simulink model "MCity_cs"  (Simulink 8.9)
settings: Solver=ode5  StartTime=0.0  StopTime=3.95  FixedStep=1/200  RelTol=1e-3
PreLoadFcn:
  | check_NUTS_defined;
  | 
  | assignin('base',['model_closed_' bdroot],false);
InitFcn:
  | PreScanExperimentInitFcn(bdroot)
StopFcn:
  | PreScanExperimentStopFcn(bdroot)
values from neighbouring files (symbols this model uses):
  d_offset = -18.15    [monocityTestLeftTurn.mat]    (also in simulation_leftTurn_PreScan.m = dl/vl*vh - 43 + R)
undefined symbols (not defined in the file or in its folder): DiscIntNeverNeededParam, warningInitialVelocity, x0
libraries: simulink x78, PreScanSimulinkLibrary x14, simulink_extras x10, PreScanUsefulBlocks x4
(part 3 of 12)

== system MCity_cs/VISUCasingLights_1_TrafficLightDoubleUS_9 ==
  CasingLights : Inport
  Demux4 : Demux  Outputs=3
  Saturation1 : Saturate  UpperLimit=1  LowerLimit=0
  Saturation2 : Saturate  UpperLimit=1  LowerLimit=0
  Saturation3 : Saturate  UpperLimit=1  LowerLimit=0
  conv_Green : Subsystem
  conv_Orange : Subsystem
  conv_Red : Subsystem
  visu_CasingGreen : Subsystem  mask(ToSensorWorld){PortName=visu_LightCasingGreen_1, PortIndex=702, PortWidth=16, TimeStep=1/200}
      mask prompts: PortName "Port Name [-]"; PortIndex "Index [-]"; PortWidth "Port Dimensions [-]"; TimeStep "Upload Period [s]"
      mask help: Sends signal(s) from Simulink to the Sensor World
      mask Help:
      | Sends signal(s) from Simulink to the Sensor World.
      | 
      | - Port Name [-]: specifies the name of the output terminal of the Simulink block.
      | - Index [-]: specifies the start position in the output vector sent to the Sensor World
      | - Port dimensions [-]: specifies the width (number of scalars) of the output port
      | - Upload period [s]: specifies the upload period (in seconds) of the port.
      mask Display: port_label('input', 1, PortName)
  visu_CasingOrange : Subsystem  mask(ToSensorWorld){PortName=visu_LightCasingOrange_1, PortIndex=718, PortWidth=16, TimeStep=1/200}
      mask prompts: PortName "Port Name [-]"; PortIndex "Index [-]"; PortWidth "Port Dimensions [-]"; TimeStep "Upload Period [s]"
      mask help: Sends signal(s) from Simulink to the Sensor World
      mask Help:
      | Sends signal(s) from Simulink to the Sensor World.
      | 
      | - Port Name [-]: specifies the name of the output terminal of the Simulink block.
      | - Index [-]: specifies the start position in the output vector sent to the Sensor World
      | - Port dimensions [-]: specifies the width (number of scalars) of the output port
      | - Upload period [s]: specifies the upload period (in seconds) of the port.
      mask Display: port_label('input', 1, PortName)
  visu_CasingRed : Subsystem  mask(ToSensorWorld){PortName=visu_LightCasingRed_1, PortIndex=734, PortWidth=16, TimeStep=1/200}
      mask prompts: PortName "Port Name [-]"; PortIndex "Index [-]"; PortWidth "Port Dimensions [-]"; TimeStep "Upload Period [s]"
      mask help: Sends signal(s) from Simulink to the Sensor World
      mask Help:
      | Sends signal(s) from Simulink to the Sensor World.
      | 
      | - Port Name [-]: specifies the name of the output terminal of the Simulink block.
      | - Index [-]: specifies the start position in the output vector sent to the Sensor World
      | - Port dimensions [-]: specifies the width (number of scalars) of the output port
      | - Upload period [s]: specifies the upload period (in seconds) of the port.
      mask Display: port_label('input', 1, PortName)
  wires:
  CasingLights/1 -> Demux4/1
  Demux4/3 -> Saturation3/1
  Demux4/2 -> Saturation2/1
  Demux4/1 -> Saturation1/1
  Saturation1/1 -> conv_Red/1(on_off)
  Saturation2/1 -> conv_Orange/1(on_off)
  Saturation3/1 -> conv_Green/1(on_off)
  conv_Red/1(RGBcolor) -> visu_CasingRed/1(Y)
  conv_Orange/1(RGBcolor) -> visu_CasingOrange/1(Y)
  conv_Green/1(RGBcolor) -> visu_CasingGreen/1(Y)

== system MCity_cs/VISUCasingLights_2_TrafficLightDoubleUS_1 ==
  CasingLights : Inport
  Demux4 : Demux  Outputs=3
  Saturation1 : Saturate  UpperLimit=1  LowerLimit=0
  Saturation2 : Saturate  UpperLimit=1  LowerLimit=0
  Saturation3 : Saturate  UpperLimit=1  LowerLimit=0
  conv_Green : Subsystem
  conv_Orange : Subsystem
  conv_Red : Subsystem
  visu_CasingGreen : Subsystem  mask(ToSensorWorld){PortName=visu_LightCasingGreen_2, PortIndex=78, PortWidth=16, TimeStep=1/200}
      mask prompts: PortName "Port Name [-]"; PortIndex "Index [-]"; PortWidth "Port Dimensions [-]"; TimeStep "Upload Period [s]"
      mask help: Sends signal(s) from Simulink to the Sensor World
      mask Help:
      | Sends signal(s) from Simulink to the Sensor World.
      | 
      | - Port Name [-]: specifies the name of the output terminal of the Simulink block.
      | - Index [-]: specifies the start position in the output vector sent to the Sensor World
      | - Port dimensions [-]: specifies the width (number of scalars) of the output port
      | - Upload period [s]: specifies the upload period (in seconds) of the port.
      mask Display: port_label('input', 1, PortName)
  visu_CasingOrange : Subsystem  mask(ToSensorWorld){PortName=visu_LightCasingOrange_2, PortIndex=94, PortWidth=16, TimeStep=1/200}
      mask prompts: PortName "Port Name [-]"; PortIndex "Index [-]"; PortWidth "Port Dimensions [-]"; TimeStep "Upload Period [s]"
      mask help: Sends signal(s) from Simulink to the Sensor World
      mask Help:
      | Sends signal(s) from Simulink to the Sensor World.
      | 
      | - Port Name [-]: specifies the name of the output terminal of the Simulink block.
      | - Index [-]: specifies the start position in the output vector sent to the Sensor World
      | - Port dimensions [-]: specifies the width (number of scalars) of the output port
      | - Upload period [s]: specifies the upload period (in seconds) of the port.
      mask Display: port_label('input', 1, PortName)
  visu_CasingRed : Subsystem  mask(ToSensorWorld){PortName=visu_LightCasingRed_2, PortIndex=110, PortWidth=16, TimeStep=1/200}
      mask prompts: PortName "Port Name [-]"; PortIndex "Index [-]"; PortWidth "Port Dimensions [-]"; TimeStep "Upload Period [s]"
      mask help: Sends signal(s) from Simulink to the Sensor World
      mask Help:
      | Sends signal(s) from Simulink to the Sensor World.
      | 
      | - Port Name [-]: specifies the name of the output terminal of the Simulink block.
      | - Index [-]: specifies the start position in the output vector sent to the Sensor World
      | - Port dimensions [-]: specifies the width (number of scalars) of the output port
      | - Upload period [s]: specifies the upload period (in seconds) of the port.
      mask Display: port_label('input', 1, PortName)
  wires:
  CasingLights/1 -> Demux4/1
  Demux4/3 -> Saturation3/1
  Demux4/2 -> Saturation2/1
  Demux4/1 -> Saturation1/1
  Saturation1/1 -> conv_Red/1(on_off)
  Saturation2/1 -> conv_Orange/1(on_off)
  Saturation3/1 -> conv_Green/1(on_off)
  conv_Red/1(RGBcolor) -> visu_CasingRed/1(Y)
  conv_Orange/1(RGBcolor) -> visu_CasingOrange/1(Y)
  conv_Green/1(RGBcolor) -> visu_CasingGreen/1(Y)

== system MCity_cs/VISUCasingLights_2_TrafficLightDoubleUS_10 ==
  CasingLights : Inport
  Demux4 : Demux  Outputs=3
  Saturation1 : Saturate  UpperLimit=1  LowerLimit=0
  Saturation2 : Saturate  UpperLimit=1  LowerLimit=0
  Saturation3 : Saturate  UpperLimit=1  LowerLimit=0
  conv_Green : Subsystem
  conv_Orange : Subsystem
  conv_Red : Subsystem
  visu_CasingGreen : Subsystem  mask(ToSensorWorld){PortName=visu_LightCasingGreen_2, PortIndex=846, PortWidth=16, TimeStep=1/200}
      mask prompts: PortName "Port Name [-]"; PortIndex "Index [-]"; PortWidth "Port Dimensions [-]"; TimeStep "Upload Period [s]"
      mask help: Sends signal(s) from Simulink to the Sensor World
      mask Help:
      | Sends signal(s) from Simulink to the Sensor World.
      | 
      | - Port Name [-]: specifies the name of the output terminal of the Simulink block.
      | - Index [-]: specifies the start position in the output vector sent to the Sensor World
      | - Port dimensions [-]: specifies the width (number of scalars) of the output port
      | - Upload period [s]: specifies the upload period (in seconds) of the port.
      mask Display: port_label('input', 1, PortName)
  visu_CasingOrange : Subsystem  mask(ToSensorWorld){PortName=visu_LightCasingOrange_2, PortIndex=862, PortWidth=16, TimeStep=1/200}
      mask prompts: PortName "Port Name [-]"; PortIndex "Index [-]"; PortWidth "Port Dimensions [-]"; TimeStep "Upload Period [s]"
      mask help: Sends signal(s) from Simulink to the Sensor World
      mask Help:
      | Sends signal(s) from Simulink to the Sensor World.
      | 
      | - Port Name [-]: specifies the name of the output terminal of the Simulink block.
      | - Index [-]: specifies the start position in the output vector sent to the Sensor World
      | - Port dimensions [-]: specifies the width (number of scalars) of the output port
      | - Upload period [s]: specifies the upload period (in seconds) of the port.
      mask Display: port_label('input', 1, PortName)
  visu_CasingRed : Subsystem  mask(ToSensorWorld){PortName=visu_LightCasingRed_2, PortIndex=878, PortWidth=16, TimeStep=1/200}
      mask prompts: PortName "Port Name [-]"; PortIndex "Index [-]"; PortWidth "Port Dimensions [-]"; TimeStep "Upload Period [s]"
      mask help: Sends signal(s) from Simulink to the Sensor World
      mask Help:
      | Sends signal(s) from Simulink to the Sensor World.
      | 
      | - Port Name [-]: specifies the name of the output terminal of the Simulink block.
      | - Index [-]: specifies the start position in the output vector sent to the Sensor World
      | - Port dimensions [-]: specifies the width (number of scalars) of the output port
      | - Upload period [s]: specifies the upload period (in seconds) of the port.
      mask Display: port_label('input', 1, PortName)
  wires:
  CasingLights/1 -> Demux4/1
  Demux4/3 -> Saturation3/1
  Demux4/2 -> Saturation2/1
  Demux4/1 -> Saturation1/1
  Saturation1/1 -> conv_Red/1(on_off)
  Saturation2/1 -> conv_Orange/1(on_off)
  Saturation3/1 -> conv_Green/1(on_off)
  conv_Red/1(RGBcolor) -> visu_CasingRed/1(Y)
  conv_Orange/1(RGBcolor) -> visu_CasingOrange/1(Y)
  conv_Green/1(RGBcolor) -> visu_CasingGreen/1(Y)

== system MCity_cs/VISUCasingLights_2_TrafficLightDoubleUS_2 ==
  CasingLights : Inport
  Demux4 : Demux  Outputs=3
  Saturation1 : Saturate  UpperLimit=1  LowerLimit=0
  Saturation2 : Saturate  UpperLimit=1  LowerLimit=0
  Saturation3 : Saturate  UpperLimit=1  LowerLimit=0
  conv_Green : Subsystem
  conv_Orange : Subsystem
  conv_Red : Subsystem
  visu_CasingGreen : Subsystem  mask(ToSensorWorld){PortName=visu_LightCasingGreen_2, PortIndex=174, PortWidth=16, TimeStep=1/200}
      mask prompts: PortName "Port Name [-]"; PortIndex "Index [-]"; PortWidth "Port Dimensions [-]"; TimeStep "Upload Period [s]"
      mask help: Sends signal(s) from Simulink to the Sensor World
      mask Help:
      | Sends signal(s) from Simulink to the Sensor World.
      | 
      | - Port Name [-]: specifies the name of the output terminal of the Simulink block.
      | - Index [-]: specifies the start position in the output vector sent to the Sensor World
      | - Port dimensions [-]: specifies the width (number of scalars) of the output port
      | - Upload period [s]: specifies the upload period (in seconds) of the port.
      mask Display: port_label('input', 1, PortName)
  visu_CasingOrange : Subsystem  mask(ToSensorWorld){PortName=visu_LightCasingOrange_2, PortIndex=190, PortWidth=16, TimeStep=1/200}
      mask prompts: PortName "Port Name [-]"; PortIndex "Index [-]"; PortWidth "Port Dimensions [-]"; TimeStep "Upload Period [s]"
      mask help: Sends signal(s) from Simulink to the Sensor World
      mask Help:
      | Sends signal(s) from Simulink to the Sensor World.
      | 
      | - Port Name [-]: specifies the name of the output terminal of the Simulink block.
      | - Index [-]: specifies the start position in the output vector sent to the Sensor World
      | - Port dimensions [-]: specifies the width (number of scalars) of the output port
      | - Upload period [s]: specifies the upload period (in seconds) of the port.
      mask Display: port_label('input', 1, PortName)
  visu_CasingRed : Subsystem  mask(ToSensorWorld){PortName=visu_LightCasingRed_2, PortIndex=206, PortWidth=16, TimeStep=1/200}
      mask prompts: PortName "Port Name [-]"; PortIndex "Index [-]"; PortWidth "Port Dimensions [-]"; TimeStep "Upload Period [s]"
      mask help: Sends signal(s) from Simulink to the Sensor World
      mask Help:
      | Sends signal(s) from Simulink to the Sensor World.
      | 
      | - Port Name [-]: specifies the name of the output terminal of the Simulink block.
      | - Index [-]: specifies the start position in the output vector sent to the Sensor World
      | - Port dimensions [-]: specifies the width (number of scalars) of the output port
      | - Upload period [s]: specifies the upload period (in seconds) of the port.
      mask Display: port_label('input', 1, PortName)
  wires:
  CasingLights/1 -> Demux4/1
  Demux4/3 -> Saturation3/1
  Demux4/2 -> Saturation2/1
  Demux4/1 -> Saturation1/1
  Saturation1/1 -> conv_Red/1(on_off)
  Saturation2/1 -> conv_Orange/1(on_off)
  Saturation3/1 -> conv_Green/1(on_off)
  conv_Red/1(RGBcolor) -> visu_CasingRed/1(Y)
  conv_Orange/1(RGBcolor) -> visu_CasingOrange/1(Y)
  conv_Green/1(RGBcolor) -> visu_CasingGreen/1(Y)

== system MCity_cs/VISUCasingLights_2_TrafficLightDoubleUS_3 ==
  CasingLights : Inport
  Demux4 : Demux  Outputs=3
  Saturation1 : Saturate  UpperLimit=1  LowerLimit=0
  Saturation2 : Saturate  UpperLimit=1  LowerLimit=0
  Saturation3 : Saturate  UpperLimit=1  LowerLimit=0
  conv_Green : Subsystem
  conv_Orange : Subsystem
  conv_Red : Subsystem
  visu_CasingGreen : Subsystem  mask(ToSensorWorld){PortName=visu_LightCasingGreen_2, PortIndex=270, PortWidth=16, TimeStep=1/200}
      mask prompts: PortName "Port Name [-]"; PortIndex "Index [-]"; PortWidth "Port Dimensions [-]"; TimeStep "Upload Period [s]"
      mask help: Sends signal(s) from Simulink to the Sensor World
      mask Help:
      | Sends signal(s) from Simulink to the Sensor World.
      | 
      | - Port Name [-]: specifies the name of the output terminal of the Simulink block.
      | - Index [-]: specifies the start position in the output vector sent to the Sensor World
      | - Port dimensions [-]: specifies the width (number of scalars) of the output port
      | - Upload period [s]: specifies the upload period (in seconds) of the port.
      mask Display: port_label('input', 1, PortName)
  visu_CasingOrange : Subsystem  mask(ToSensorWorld){PortName=visu_LightCasingOrange_2, PortIndex=286, PortWidth=16, TimeStep=1/200}
      mask prompts: PortName "Port Name [-]"; PortIndex "Index [-]"; PortWidth "Port Dimensions [-]"; TimeStep "Upload Period [s]"
      mask help: Sends signal(s) from Simulink to the Sensor World
      mask Help:
      | Sends signal(s) from Simulink to the Sensor World.
      | 
      | - Port Name [-]: specifies the name of the output terminal of the Simulink block.
      | - Index [-]: specifies the start position in the output vector sent to the Sensor World
      | - Port dimensions [-]: specifies the width (number of scalars) of the output port
      | - Upload period [s]: specifies the upload period (in seconds) of the port.
      mask Display: port_label('input', 1, PortName)
  visu_CasingRed : Subsystem  mask(ToSensorWorld){PortName=visu_LightCasingRed_2, PortIndex=302, PortWidth=16, TimeStep=1/200}
      mask prompts: PortName "Port Name [-]"; PortIndex "Index [-]"; PortWidth "Port Dimensions [-]"; TimeStep "Upload Period [s]"
      mask help: Sends signal(s) from Simulink to the Sensor World
      mask Help:
      | Sends signal(s) from Simulink to the Sensor World.
      | 
      | - Port Name [-]: specifies the name of the output terminal of the Simulink block.
      | - Index [-]: specifies the start position in the output vector sent to the Sensor World
      | - Port dimensions [-]: specifies the width (number of scalars) of the output port
      | - Upload period [s]: specifies the upload period (in seconds) of the port.
      mask Display: port_label('input', 1, PortName)
  wires:
  CasingLights/1 -> Demux4/1
  Demux4/3 -> Saturation3/1
  Demux4/2 -> Saturation2/1
  Demux4/1 -> Saturation1/1
  Saturation1/1 -> conv_Red/1(on_off)
  Saturation2/1 -> conv_Orange/1(on_off)
  Saturation3/1 -> conv_Green/1(on_off)
  conv_Red/1(RGBcolor) -> visu_CasingRed/1(Y)
  conv_Orange/1(RGBcolor) -> visu_CasingOrange/1(Y)
  conv_Green/1(RGBcolor) -> visu_CasingGreen/1(Y)

== system MCity_cs/VISUCasingLights_2_TrafficLightDoubleUS_4 ==
  CasingLights : Inport
  Demux4 : Demux  Outputs=3
  Saturation1 : Saturate  UpperLimit=1  LowerLimit=0
  Saturation2 : Saturate  UpperLimit=1  LowerLimit=0
  Saturation3 : Saturate  UpperLimit=1  LowerLimit=0
  conv_Green : Subsystem
  conv_Orange : Subsystem
  conv_Red : Subsystem
  visu_CasingGreen : Subsystem  mask(ToSensorWorld){PortName=visu_LightCasingGreen_2, PortIndex=366, PortWidth=16, TimeStep=1/200}
      mask prompts: PortName "Port Name [-]"; PortIndex "Index [-]"; PortWidth "Port Dimensions [-]"; TimeStep "Upload Period [s]"
      mask help: Sends signal(s) from Simulink to the Sensor World
      mask Help:
      | Sends signal(s) from Simulink to the Sensor World.
      | 
      | - Port Name [-]: specifies the name of the output terminal of the Simulink block.
      | - Index [-]: specifies the start position in the output vector sent to the Sensor World
      | - Port dimensions [-]: specifies the width (number of scalars) of the output port
      | - Upload period [s]: specifies the upload period (in seconds) of the port.
      mask Display: port_label('input', 1, PortName)
  visu_CasingOrange : Subsystem  mask(ToSensorWorld){PortName=visu_LightCasingOrange_2, PortIndex=382, PortWidth=16, TimeStep=1/200}
      mask prompts: PortName "Port Name [-]"; PortIndex "Index [-]"; PortWidth "Port Dimensions [-]"; TimeStep "Upload Period [s]"
      mask help: Sends signal(s) from Simulink to the Sensor World
      mask Help:
      | Sends signal(s) from Simulink to the Sensor World.
      | 
      | - Port Name [-]: specifies the name of the output terminal of the Simulink block.
      | - Index [-]: specifies the start position in the output vector sent to the Sensor World
      | - Port dimensions [-]: specifies the width (number of scalars) of the output port
      | - Upload period [s]: specifies the upload period (in seconds) of the port.
      mask Display: port_label('input', 1, PortName)
  visu_CasingRed : Subsystem  mask(ToSensorWorld){PortName=visu_LightCasingRed_2, PortIndex=398, PortWidth=16, TimeStep=1/200}
      mask prompts: PortName "Port Name [-]"; PortIndex "Index [-]"; PortWidth "Port Dimensions [-]"; TimeStep "Upload Period [s]"
      mask help: Sends signal(s) from Simulink to the Sensor World
      mask Help:
      | Sends signal(s) from Simulink to the Sensor World.
      | 
      | - Port Name [-]: specifies the name of the output terminal of the Simulink block.
      | - Index [-]: specifies the start position in the output vector sent to the Sensor World
      | - Port dimensions [-]: specifies the width (number of scalars) of the output port
      | - Upload period [s]: specifies the upload period (in seconds) of the port.
      mask Display: port_label('input', 1, PortName)
  wires:
  CasingLights/1 -> Demux4/1
  Demux4/3 -> Saturation3/1
  Demux4/2 -> Saturation2/1
  Demux4/1 -> Saturation1/1
  Saturation1/1 -> conv_Red/1(on_off)
  Saturation2/1 -> conv_Orange/1(on_off)
  Saturation3/1 -> conv_Green/1(on_off)
  conv_Red/1(RGBcolor) -> visu_CasingRed/1(Y)
  conv_Orange/1(RGBcolor) -> visu_CasingOrange/1(Y)
  conv_Green/1(RGBcolor) -> visu_CasingGreen/1(Y)

== system MCity_cs/VISUCasingLights_2_TrafficLightDoubleUS_5 ==
  CasingLights : Inport
  Demux4 : Demux  Outputs=3
  Saturation1 : Saturate  UpperLimit=1  LowerLimit=0
  Saturation2 : Saturate  UpperLimit=1  LowerLimit=0
  Saturation3 : Saturate  UpperLimit=1  LowerLimit=0
  conv_Green : Subsystem
  conv_Orange : Subsystem
  conv_Red : Subsystem
  visu_CasingGreen : Subsystem  mask(ToSensorWorld){PortName=visu_LightCasingGreen_2, PortIndex=942, PortWidth=16, TimeStep=1/200}
      mask prompts: PortName "Port Name [-]"; PortIndex "Index [-]"; PortWidth "Port Dimensions [-]"; TimeStep "Upload Period [s]"
      mask help: Sends signal(s) from Simulink to the Sensor World
      mask Help:
      | Sends signal(s) from Simulink to the Sensor World.
      | 
      | - Port Name [-]: specifies the name of the output terminal of the Simulink block.
      | - Index [-]: specifies the start position in the output vector sent to the Sensor World
      | - Port dimensions [-]: specifies the width (number of scalars) of the output port
      | - Upload period [s]: specifies the upload period (in seconds) of the port.
      mask Display: port_label('input', 1, PortName)
  visu_CasingOrange : Subsystem  mask(ToSensorWorld){PortName=visu_LightCasingOrange_2, PortIndex=958, PortWidth=16, TimeStep=1/200}
      mask prompts: PortName "Port Name [-]"; PortIndex "Index [-]"; PortWidth "Port Dimensions [-]"; TimeStep "Upload Period [s]"
      mask help: Sends signal(s) from Simulink to the Sensor World
      mask Help:
      | Sends signal(s) from Simulink to the Sensor World.
      | 
      | - Port Name [-]: specifies the name of the output terminal of the Simulink block.
      | - Index [-]: specifies the start position in the output vector sent to the Sensor World
      | - Port dimensions [-]: specifies the width (number of scalars) of the output port
      | - Upload period [s]: specifies the upload period (in seconds) of the port.
      mask Display: port_label('input', 1, PortName)
  visu_CasingRed : Subsystem  mask(ToSensorWorld){PortName=visu_LightCasingRed_2, PortIndex=974, PortWidth=16, TimeStep=1/200}
      mask prompts: PortName "Port Name [-]"; PortIndex "Index [-]"; PortWidth "Port Dimensions [-]"; TimeStep "Upload Period [s]"
      mask help: Sends signal(s) from Simulink to the Sensor World
      mask Help:
      | Sends signal(s) from Simulink to the Sensor World.
      | 
      | - Port Name [-]: specifies the name of the output terminal of the Simulink block.
      | - Index [-]: specifies the start position in the output vector sent to the Sensor World
      | - Port dimensions [-]: specifies the width (number of scalars) of the output port
      | - Upload period [s]: specifies the upload period (in seconds) of the port.
      mask Display: port_label('input', 1, PortName)
  wires:
  CasingLights/1 -> Demux4/1
  Demux4/3 -> Saturation3/1
  Demux4/2 -> Saturation2/1
  Demux4/1 -> Saturation1/1
  Saturation1/1 -> conv_Red/1(on_off)
  Saturation2/1 -> conv_Orange/1(on_off)
  Saturation3/1 -> conv_Green/1(on_off)
  conv_Red/1(RGBcolor) -> visu_CasingRed/1(Y)
  conv_Orange/1(RGBcolor) -> visu_CasingOrange/1(Y)
  conv_Green/1(RGBcolor) -> visu_CasingGreen/1(Y)

== system MCity_cs/VISUCasingLights_2_TrafficLightDoubleUS_6 ==
  CasingLights : Inport
  Demux4 : Demux  Outputs=3
  Saturation1 : Saturate  UpperLimit=1  LowerLimit=0
  Saturation2 : Saturate  UpperLimit=1  LowerLimit=0
  Saturation3 : Saturate  UpperLimit=1  LowerLimit=0
  conv_Green : Subsystem
  conv_Orange : Subsystem
  conv_Red : Subsystem
  visu_CasingGreen : Subsystem  mask(ToSensorWorld){PortName=visu_LightCasingGreen_2, PortIndex=462, PortWidth=16, TimeStep=1/200}
      mask prompts: PortName "Port Name [-]"; PortIndex "Index [-]"; PortWidth "Port Dimensions [-]"; TimeStep "Upload Period [s]"
      mask help: Sends signal(s) from Simulink to the Sensor World
      mask Help:
      | Sends signal(s) from Simulink to the Sensor World.
      | 
      | - Port Name [-]: specifies the name of the output terminal of the Simulink block.
      | - Index [-]: specifies the start position in the output vector sent to the Sensor World
      | - Port dimensions [-]: specifies the width (number of scalars) of the output port
      | - Upload period [s]: specifies the upload period (in seconds) of the port.
      mask Display: port_label('input', 1, PortName)
  visu_CasingOrange : Subsystem  mask(ToSensorWorld){PortName=visu_LightCasingOrange_2, PortIndex=478, PortWidth=16, TimeStep=1/200}
      mask prompts: PortName "Port Name [-]"; PortIndex "Index [-]"; PortWidth "Port Dimensions [-]"; TimeStep "Upload Period [s]"
      mask help: Sends signal(s) from Simulink to the Sensor World
      mask Help:
      | Sends signal(s) from Simulink to the Sensor World.
      | 
      | - Port Name [-]: specifies the name of the output terminal of the Simulink block.
      | - Index [-]: specifies the start position in the output vector sent to the Sensor World
      | - Port dimensions [-]: specifies the width (number of scalars) of the output port
      | - Upload period [s]: specifies the upload period (in seconds) of the port.
      mask Display: port_label('input', 1, PortName)
  visu_CasingRed : Subsystem  mask(ToSensorWorld){PortName=visu_LightCasingRed_2, PortIndex=494, PortWidth=16, TimeStep=1/200}
      mask prompts: PortName "Port Name [-]"; PortIndex "Index [-]"; PortWidth "Port Dimensions [-]"; TimeStep "Upload Period [s]"
      mask help: Sends signal(s) from Simulink to the Sensor World
      mask Help:
      | Sends signal(s) from Simulink to the Sensor World.
      | 
      | - Port Name [-]: specifies the name of the output terminal of the Simulink block.
      | - Index [-]: specifies the start position in the output vector sent to the Sensor World
      | - Port dimensions [-]: specifies the width (number of scalars) of the output port
      | - Upload period [s]: specifies the upload period (in seconds) of the port.
      mask Display: port_label('input', 1, PortName)
  wires:
  CasingLights/1 -> Demux4/1
  Demux4/3 -> Saturation3/1
  Demux4/2 -> Saturation2/1
  Demux4/1 -> Saturation1/1
  Saturation1/1 -> conv_Red/1(on_off)
  Saturation2/1 -> conv_Orange/1(on_off)
  Saturation3/1 -> conv_Green/1(on_off)
  conv_Red/1(RGBcolor) -> visu_CasingRed/1(Y)
  conv_Orange/1(RGBcolor) -> visu_CasingOrange/1(Y)
  conv_Green/1(RGBcolor) -> visu_CasingGreen/1(Y)

== system MCity_cs/VISUCasingLights_2_TrafficLightDoubleUS_7 ==
  CasingLights : Inport
  Demux4 : Demux  Outputs=3
  Saturation1 : Saturate  UpperLimit=1  LowerLimit=0
  Saturation2 : Saturate  UpperLimit=1  LowerLimit=0
  Saturation3 : Saturate  UpperLimit=1  LowerLimit=0
  conv_Green : Subsystem
  conv_Orange : Subsystem
  conv_Red : Subsystem
  visu_CasingGreen : Subsystem  mask(ToSensorWorld){PortName=visu_LightCasingGreen_2, PortIndex=654, PortWidth=16, TimeStep=1/200}
      mask prompts: PortName "Port Name [-]"; PortIndex "Index [-]"; PortWidth "Port Dimensions [-]"; TimeStep "Upload Period [s]"
      mask help: Sends signal(s) from Simulink to the Sensor World
      mask Help:
      | Sends signal(s) from Simulink to the Sensor World.
      | 
      | - Port Name [-]: specifies the name of the output terminal of the Simulink block.
      | - Index [-]: specifies the start position in the output vector sent to the Sensor World
      | - Port dimensions [-]: specifies the width (number of scalars) of the output port
      | - Upload period [s]: specifies the upload period (in seconds) of the port.
      mask Display: port_label('input', 1, PortName)
  visu_CasingOrange : Subsystem  mask(ToSensorWorld){PortName=visu_LightCasingOrange_2, PortIndex=670, PortWidth=16, TimeStep=1/200}
      mask prompts: PortName "Port Name [-]"; PortIndex "Index [-]"; PortWidth "Port Dimensions [-]"; TimeStep "Upload Period [s]"
      mask help: Sends signal(s) from Simulink to the Sensor World
      mask Help:
      | Sends signal(s) from Simulink to the Sensor World.
      | 
      | - Port Name [-]: specifies the name of the output terminal of the Simulink block.
      | - Index [-]: specifies the start position in the output vector sent to the Sensor World
      | - Port dimensions [-]: specifies the width (number of scalars) of the output port
      | - Upload period [s]: specifies the upload period (in seconds) of the port.
      mask Display: port_label('input', 1, PortName)
  visu_CasingRed : Subsystem  mask(ToSensorWorld){PortName=visu_LightCasingRed_2, PortIndex=686, PortWidth=16, TimeStep=1/200}
      mask prompts: PortName "Port Name [-]"; PortIndex "Index [-]"; PortWidth "Port Dimensions [-]"; TimeStep "Upload Period [s]"
      mask help: Sends signal(s) from Simulink to the Sensor World
      mask Help:
      | Sends signal(s) from Simulink to the Sensor World.
      | 
      | - Port Name [-]: specifies the name of the output terminal of the Simulink block.
      | - Index [-]: specifies the start position in the output vector sent to the Sensor World
      | - Port dimensions [-]: specifies the width (number of scalars) of the output port
      | - Upload period [s]: specifies the upload period (in seconds) of the port.
      mask Display: port_label('input', 1, PortName)
  wires:
  CasingLights/1 -> Demux4/1
  Demux4/3 -> Saturation3/1
  Demux4/2 -> Saturation2/1
  Demux4/1 -> Saturation1/1
  Saturation1/1 -> conv_Red/1(on_off)
  Saturation2/1 -> conv_Orange/1(on_off)
  Saturation3/1 -> conv_Green/1(on_off)
  conv_Red/1(RGBcolor) -> visu_CasingRed/1(Y)
  conv_Orange/1(RGBcolor) -> visu_CasingOrange/1(Y)
  conv_Green/1(RGBcolor) -> visu_CasingGreen/1(Y)

== system MCity_cs/VISUCasingLights_2_TrafficLightDoubleUS_8 ==
  CasingLights : Inport
  Demux4 : Demux  Outputs=3
  Saturation1 : Saturate  UpperLimit=1  LowerLimit=0
  Saturation2 : Saturate  UpperLimit=1  LowerLimit=0
  Saturation3 : Saturate  UpperLimit=1  LowerLimit=0
  conv_Green : Subsystem
  conv_Orange : Subsystem
  conv_Red : Subsystem
  visu_CasingGreen : Subsystem  mask(ToSensorWorld){PortName=visu_LightCasingGreen_2, PortIndex=1038, PortWidth=16, TimeStep=1/200}
      mask prompts: PortName "Port Name [-]"; PortIndex "Index [-]"; PortWidth "Port Dimensions [-]"; TimeStep "Upload Period [s]"
      mask help: Sends signal(s) from Simulink to the Sensor World
      mask Help:
      | Sends signal(s) from Simulink to the Sensor World.
      | 
      | - Port Name [-]: specifies the name of the output terminal of the Simulink block.
      | - Index [-]: specifies the start position in the output vector sent to the Sensor World
      | - Port dimensions [-]: specifies the width (number of scalars) of the output port
      | - Upload period [s]: specifies the upload period (in seconds) of the port.
      mask Display: port_label('input', 1, PortName)
  visu_CasingOrange : Subsystem  mask(ToSensorWorld){PortName=visu_LightCasingOrange_2, PortIndex=1054, PortWidth=16, TimeStep=1/200}
      mask prompts: PortName "Port Name [-]"; PortIndex "Index [-]"; PortWidth "Port Dimensions [-]"; TimeStep "Upload Period [s]"
      mask help: Sends signal(s) from Simulink to the Sensor World
      mask Help:
      | Sends signal(s) from Simulink to the Sensor World.
      | 
      | - Port Name [-]: specifies the name of the output terminal of the Simulink block.
      | - Index [-]: specifies the start position in the output vector sent to the Sensor World
      | - Port dimensions [-]: specifies the width (number of scalars) of the output port
      | - Upload period [s]: specifies the upload period (in seconds) of the port.
      mask Display: port_label('input', 1, PortName)
  visu_CasingRed : Subsystem  mask(ToSensorWorld){PortName=visu_LightCasingRed_2, PortIndex=1070, PortWidth=16, TimeStep=1/200}
      mask prompts: PortName "Port Name [-]"; PortIndex "Index [-]"; PortWidth "Port Dimensions [-]"; TimeStep "Upload Period [s]"
      mask help: Sends signal(s) from Simulink to the Sensor World
      mask Help:
      | Sends signal(s) from Simulink to the Sensor World.
      | 
      | - Port Name [-]: specifies the name of the output terminal of the Simulink block.
      | - Index [-]: specifies the start position in the output vector sent to the Sensor World
      | - Port dimensions [-]: specifies the width (number of scalars) of the output port
      | - Upload period [s]: specifies the upload period (in seconds) of the port.
      mask Display: port_label('input', 1, PortName)
  wires:
  CasingLights/1 -> Demux4/1
  Demux4/3 -> Saturation3/1
  Demux4/2 -> Saturation2/1
  Demux4/1 -> Saturation1/1
  Saturation1/1 -> conv_Red/1(on_off)
  Saturation2/1 -> conv_Orange/1(on_off)
  Saturation3/1 -> conv_Green/1(on_off)
  conv_Red/1(RGBcolor) -> visu_CasingRed/1(Y)
  conv_Orange/1(RGBcolor) -> visu_CasingOrange/1(Y)
  conv_Green/1(RGBcolor) -> visu_CasingGreen/1(Y)

== system MCity_cs/VISUCasingLights_2_TrafficLightDoubleUS_9 ==
  CasingLights : Inport
  Demux4 : Demux  Outputs=3
  Saturation1 : Saturate  UpperLimit=1  LowerLimit=0
  Saturation2 : Saturate  UpperLimit=1  LowerLimit=0
  Saturation3 : Saturate  UpperLimit=1  LowerLimit=0
  conv_Green : Subsystem
  conv_Orange : Subsystem
  conv_Red : Subsystem
  visu_CasingGreen : Subsystem  mask(ToSensorWorld){PortName=visu_LightCasingGreen_2, PortIndex=750, PortWidth=16, TimeStep=1/200}
      mask prompts: PortName "Port Name [-]"; PortIndex "Index [-]"; PortWidth "Port Dimensions [-]"; TimeStep "Upload Period [s]"
      mask help: Sends signal(s) from Simulink to the Sensor World
      mask Help:
      | Sends signal(s) from Simulink to the Sensor World.
      | 
      | - Port Name [-]: specifies the name of the output terminal of the Simulink block.
      | - Index [-]: specifies the start position in the output vector sent to the Sensor World
      | - Port dimensions [-]: specifies the width (number of scalars) of the output port
      | - Upload period [s]: specifies the upload period (in seconds) of the port.
      mask Display: port_label('input', 1, PortName)
  visu_CasingOrange : Subsystem  mask(ToSensorWorld){PortName=visu_LightCasingOrange_2, PortIndex=766, PortWidth=16, TimeStep=1/200}
      mask prompts: PortName "Port Name [-]"; PortIndex "Index [-]"; PortWidth "Port Dimensions [-]"; TimeStep "Upload Period [s]"
      mask help: Sends signal(s) from Simulink to the Sensor World
      mask Help:
      | Sends signal(s) from Simulink to the Sensor World.
      | 
      | - Port Name [-]: specifies the name of the output terminal of the Simulink block.
      | - Index [-]: specifies the start position in the output vector sent to the Sensor World
      | - Port dimensions [-]: specifies the width (number of scalars) of the output port
      | - Upload period [s]: specifies the upload period (in seconds) of the port.
      mask Display: port_label('input', 1, PortName)
  visu_CasingRed : Subsystem  mask(ToSensorWorld){PortName=visu_LightCasingRed_2, PortIndex=782, PortWidth=16, TimeStep=1/200}
      mask prompts: PortName "Port Name [-]"; PortIndex "Index [-]"; PortWidth "Port Dimensions [-]"; TimeStep "Upload Period [s]"
      mask help: Sends signal(s) from Simulink to the Sensor World
      mask Help:
      | Sends signal(s) from Simulink to the Sensor World.
      | 
      | - Port Name [-]: specifies the name of the output terminal of the Simulink block.
      | - Index [-]: specifies the start position in the output vector sent to the Sensor World
      | - Port dimensions [-]: specifies the width (number of scalars) of the output port
      | - Upload period [s]: specifies the upload period (in seconds) of the port.
      mask Display: port_label('input', 1, PortName)
  wires:
  CasingLights/1 -> Demux4/1
  Demux4/3 -> Saturation3/1
  Demux4/2 -> Saturation2/1
  Demux4/1 -> Saturation1/1
  Saturation1/1 -> conv_Red/1(on_off)
  Saturation2/1 -> conv_Orange/1(on_off)
  Saturation3/1 -> conv_Green/1(on_off)
  conv_Red/1(RGBcolor) -> visu_CasingRed/1(Y)
  conv_Orange/1(RGBcolor) -> visu_CasingOrange/1(Y)
  conv_Green/1(RGBcolor) -> visu_CasingGreen/1(Y)

== system MCity_cs/VISUCasingLights_TrafficLightSingleUS_1 ==
  CasingLights : Inport
  Demux4 : Demux  Outputs=3
  Saturation1 : Saturate  UpperLimit=1  LowerLimit=0
  Saturation2 : Saturate  UpperLimit=1  LowerLimit=0
  Saturation3 : Saturate  UpperLimit=1  LowerLimit=0
  conv_Green : Subsystem
  conv_Orange : Subsystem
  conv_Red : Subsystem
  visu_CasingGreen : Subsystem  mask(ToSensorWorld){PortName=visu_LightCasingGreen_0, PortIndex=510, PortWidth=16, TimeStep=1/200}
      mask prompts: PortName "Port Name [-]"; PortIndex "Index [-]"; PortWidth "Port Dimensions [-]"; TimeStep "Upload Period [s]"
      mask help: Sends signal(s) from Simulink to the Sensor World
      mask Help:
      | Sends signal(s) from Simulink to the Sensor World.
      | 
      | - Port Name [-]: specifies the name of the output terminal of the Simulink block.
      | - Index [-]: specifies the start position in the output vector sent to the Sensor World
      | - Port dimensions [-]: specifies the width (number of scalars) of the output port
      | - Upload period [s]: specifies the upload period (in seconds) of the port.
      mask Display: port_label('input', 1, PortName)
  visu_CasingOrange : Subsystem  mask(ToSensorWorld){PortName=visu_LightCasingOrange_0, PortIndex=526, PortWidth=16, TimeStep=1/200}
      mask prompts: PortName "Port Name [-]"; PortIndex "Index [-]"; PortWidth "Port Dimensions [-]"; TimeStep "Upload Period [s]"
      mask help: Sends signal(s) from Simulink to the Sensor World
      mask Help:
      | Sends signal(s) from Simulink to the Sensor World.
      | 
      | - Port Name [-]: specifies the name of the output terminal of the Simulink block.
      | - Index [-]: specifies the start position in the output vector sent to the Sensor World
      | - Port dimensions [-]: specifies the width (number of scalars) of the output port
      | - Upload period [s]: specifies the upload period (in seconds) of the port.
      mask Display: port_label('input', 1, PortName)
  visu_CasingRed : Subsystem  mask(ToSensorWorld){PortName=visu_LightCasingRed_0, PortIndex=542, PortWidth=16, TimeStep=1/200}
      mask prompts: PortName "Port Name [-]"; PortIndex "Index [-]"; PortWidth "Port Dimensions [-]"; TimeStep "Upload Period [s]"
      mask help: Sends signal(s) from Simulink to the Sensor World
      mask Help:
      | Sends signal(s) from Simulink to the Sensor World.
      | 
      | - Port Name [-]: specifies the name of the output terminal of the Simulink block.
      | - Index [-]: specifies the start position in the output vector sent to the Sensor World
      | - Port dimensions [-]: specifies the width (number of scalars) of the output port
      | - Upload period [s]: specifies the upload period (in seconds) of the port.
      mask Display: port_label('input', 1, PortName)
  wires:
  CasingLights/1 -> Demux4/1
  Demux4/3 -> Saturation3/1
  Demux4/2 -> Saturation2/1
  Demux4/1 -> Saturation1/1
  Saturation1/1 -> conv_Red/1(on_off)
  Saturation2/1 -> conv_Orange/1(on_off)
  Saturation3/1 -> conv_Green/1(on_off)
  conv_Red/1(RGBcolor) -> visu_CasingRed/1(Y)
  conv_Orange/1(RGBcolor) -> visu_CasingOrange/1(Y)
  conv_Green/1(RGBcolor) -> visu_CasingGreen/1(Y)

== system MCity_cs/VISUCasingLights_TrafficLightSingleUS_2 ==
  CasingLights : Inport
  Demux4 : Demux  Outputs=3
  Saturation1 : Saturate  UpperLimit=1  LowerLimit=0
  Saturation2 : Saturate  UpperLimit=1  LowerLimit=0
  Saturation3 : Saturate  UpperLimit=1  LowerLimit=0
  conv_Green : Subsystem
  conv_Orange : Subsystem
  conv_Red : Subsystem
  visu_CasingGreen : Subsystem  mask(ToSensorWorld){PortName=visu_LightCasingGreen_0, PortIndex=558, PortWidth=16, TimeStep=1/200}
      mask prompts: PortName "Port Name [-]"; PortIndex "Index [-]"; PortWidth "Port Dimensions [-]"; TimeStep "Upload Period [s]"
      mask help: Sends signal(s) from Simulink to the Sensor World
      mask Help:
      | Sends signal(s) from Simulink to the Sensor World.
      | 
      | - Port Name [-]: specifies the name of the output terminal of the Simulink block.
      | - Index [-]: specifies the start position in the output vector sent to the Sensor World
      | - Port dimensions [-]: specifies the width (number of scalars) of the output port
      | - Upload period [s]: specifies the upload period (in seconds) of the port.
      mask Display: port_label('input', 1, PortName)
  visu_CasingOrange : Subsystem  mask(ToSensorWorld){PortName=visu_LightCasingOrange_0, PortIndex=574, PortWidth=16, TimeStep=1/200}
      mask prompts: PortName "Port Name [-]"; PortIndex "Index [-]"; PortWidth "Port Dimensions [-]"; TimeStep "Upload Period [s]"
      mask help: Sends signal(s) from Simulink to the Sensor World
      mask Help:
      | Sends signal(s) from Simulink to the Sensor World.
      | 
      | - Port Name [-]: specifies the name of the output terminal of the Simulink block.
      | - Index [-]: specifies the start position in the output vector sent to the Sensor World
      | - Port dimensions [-]: specifies the width (number of scalars) of the output port
      | - Upload period [s]: specifies the upload period (in seconds) of the port.
      mask Display: port_label('input', 1, PortName)
  visu_CasingRed : Subsystem  mask(ToSensorWorld){PortName=visu_LightCasingRed_0, PortIndex=590, PortWidth=16, TimeStep=1/200}
      mask prompts: PortName "Port Name [-]"; PortIndex "Index [-]"; PortWidth "Port Dimensions [-]"; TimeStep "Upload Period [s]"
      mask help: Sends signal(s) from Simulink to the Sensor World
      mask Help:
      | Sends signal(s) from Simulink to the Sensor World.
      | 
      | - Port Name [-]: specifies the name of the output terminal of the Simulink block.
      | - Index [-]: specifies the start position in the output vector sent to the Sensor World
      | - Port dimensions [-]: specifies the width (number of scalars) of the output port
      | - Upload period [s]: specifies the upload period (in seconds) of the port.
      mask Display: port_label('input', 1, PortName)
  wires:
  CasingLights/1 -> Demux4/1
  Demux4/3 -> Saturation3/1
  Demux4/2 -> Saturation2/1
  Demux4/1 -> Saturation1/1
  Saturation1/1 -> conv_Red/1(on_off)
  Saturation2/1 -> conv_Orange/1(on_off)
  Saturation3/1 -> conv_Green/1(on_off)
  conv_Red/1(RGBcolor) -> visu_CasingRed/1(Y)
  conv_Orange/1(RGBcolor) -> visu_CasingOrange/1(Y)
  conv_Green/1(RGBcolor) -> visu_CasingGreen/1(Y)

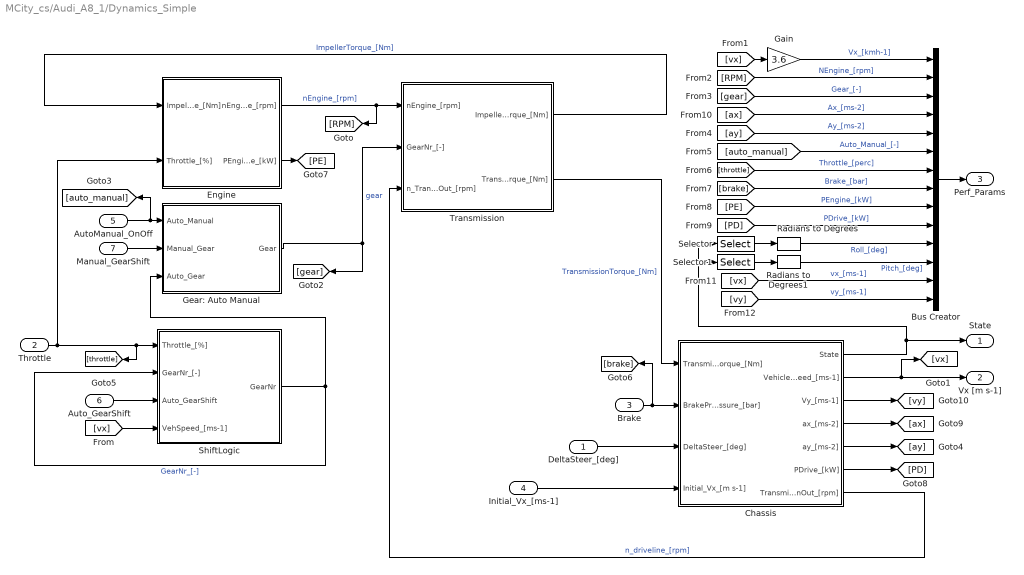
== system MCity_cs/Audi_A8_1/Dynamics_Simple ==
  DeltaSteer_[deg] : Inport
  Throttle : Inport  Port=2
  Brake : Inport  Port=3
  Initial_Vx_[ms-1] : Inport  Port=4
  AutoManual_OnOff : Inport  Port=5
  Auto_GearShift : Inport  Port=6
  Manual_GearShift : Inport  Port=7
  Bus Creator : BusCreator  Inputs=14
  Chassis : Subsystem
      mask Display: image(imread('Chassis.png'));
  Engine : Subsystem
      mask Display: image(imread('Engine.png'));
  Gain : Gain  Gain=3.6
  Gear: Auto Manual : Subsystem
  Radians to Degrees : simulink_extras/Transformations/Radians to Degrees
  Radians to Degrees1 : simulink_extras/Transformations/Radians to Degrees
  Selector : Selector  InputPortWidth=9  IndexOptions=Index vector (dialog)  Indices=7  OutputSizes=1
  Selector1 : Selector  InputPortWidth=9  IndexOptions=Index vector (dialog)  Indices=8  OutputSizes=1
  ShiftLogic : Subsystem
      mask Display: image(imread('Gearshift.png'));
  Transmission : Subsystem
      mask Display: image(imread('Transmission.png'));
  State : Outport
  Vx [m s-1] : Outport  Port=2
  Perf_Params : Outport  Port=3
  wires:
  [vy] -> Bus Creator/14  "vy_[ms-1]"
  [vx] -> Bus Creator/13  "vx_[ms-1]"
  Chassis/7(TransmissionOut_[rpm]) -> Transmission/3(n_TransmissionOut_[rpm])  "n_driveline_[rpm]"
  Chassis/6(PDrive_[kW]) -> [PD]
  Chassis/5(ay_[ms-2]) -> [ay]
  Chassis/4(ax_[ms-2]) -> [ax]
  Chassis/3(Vy_[ms-1]) -> [vy]
  [vx] -> ShiftLogic/4(VehSpeed_[ms-1])
  Gear: Auto Manual/1(Gear) -> Transmission/2(GearNr_[-]), [gear]  "gear"
  Manual_GearShift/1 -> Gear: Auto Manual/2(Manual_Gear)
  AutoManual_OnOff/1 -> Gear: Auto Manual/1(Auto_Manual), [auto_manual]
  Chassis/2(VehicleSpeed_[ms-1]) -> [vx], Vx [m s-1]/1
  Auto_GearShift/1 -> ShiftLogic/3(Auto_GearShift)
  Throttle/1 -> Engine/2(Throttle_[%]), ShiftLogic/1(Throttle_[%]), [throttle]
  Initial_Vx_[ms-1]/1 -> Chassis/4(Initial_Vx_[m s-1])
  DeltaSteer_[deg]/1 -> Chassis/3(DeltaSteer_[deg])
  Chassis/1(State) -> State/1, Selector/1, Selector1/1
  Brake/1 -> [brake], Chassis/2(BrakePressure_[bar])
  Engine/1(nEngine_[rpm]) -> [RPM], Transmission/1(nEngine_[rpm])  "nEngine_[rpm]"
  ShiftLogic/1(GearNr) -> Gear: Auto Manual/3(Auto_Gear), ShiftLogic/2(GearNr_[-])  "GearNr_[-]"
  Transmission/2(TransmissionTorque_[Nm]) -> Chassis/1(TransmissionTorque_[Nm])  "TransmissionTorque_[Nm]"
  Transmission/1(ImpellerTorque_[Nm]) -> Engine/1(ImpellerTorque_[Nm])  "ImpellerTorque_[Nm]"
  Gain/1 -> Bus Creator/1  "Vx_[kmh-1]"
  [RPM] -> Bus Creator/2  "NEngine_[rpm]"
  [gear] -> Bus Creator/3  "Gear_[-]"
  [ay] -> Bus Creator/5  "Ay_[ms-2]"
  [auto_manual] -> Bus Creator/6  "Auto_Manual_[-]"
  [throttle] -> Bus Creator/7  "Throttle_[perc]"
  [brake] -> Bus Creator/8  "Brake_[bar]"
  Engine/2(PEngine_[kW]) -> [PE]
  Bus Creator/1 -> Perf_Params/1
  [PE] -> Bus Creator/9  "PEngine_[kW]"
  Radians to Degrees/1 -> Bus Creator/11  "Roll_[deg]"
  Radians to Degrees1/1 -> Bus Creator/12  "Pitch_[deg]"
  [PD] -> Bus Creator/10  "PDrive_[kW]"
  Selector/1 -> Radians to Degrees/1
  Selector1/1 -> Radians to Degrees1/1
  [vx] -> Gain/1
  [ax] -> Bus Creator/4  "Ax_[ms-2]"

== system MCity_cs/Audi_A8_1/PathFollower_Preview_1 ==
  TrajOffset x,y,Y [m,m,deg] : Inport
  ActorOffset_Left(+) / Right(-) [m] : Inport  Port=2
  position x,y,Y [m,m,deg] : Inport  Port=3
  Initial Velocity [m/s] : Inport  Port=4
  Desired Velocity [m/s] : Inport  Port=5
  velocity [m/s] : Inport  Port=6
  vx [m/s] : Inport  Port=7
  vy [m/s] : Inport  Port=8
  Yaw rate [deg/s] : Inport  Port=9
  CorneringStiffness_Tyres_Front [N/rad] : Inport  Port=10
  CorneringStiffness_Tyres_Rear [N/rad] : Inport  Port=11
  steering_ratio[-] : Inport  Port=12
  LateralController : Subsystem
  LongitudinalController : Subsystem
  delta_steerwheel [deg] : Outport
  throttle [%] : Outport  Port=2
  brake pressure [bar] : Outport  Port=3
  v0 [m/s] : Outport  Port=4
  Auto_GearShift : Outport  Port=5
  Actor/Traj_distance [m] : Outport  Port=6
  Actor/Traj_angle [deg] : Outport  Port=7
  wires:
  LateralController/3(delta_steerwheel [deg]) -> delta_steerwheel [deg]/1
  steering_ratio[-]/1 -> LateralController/9(steering_ratio[-])
  CorneringStiffness_Tyres_Rear [N/rad]/1 -> LateralController/8(CorneringStiffness_Tyres_Rear [N/rad])
  CorneringStiffness_Tyres_Front [N/rad]/1 -> LateralController/7(CorneringStiffness_Tyres_Front [N/rad])
  Yaw rate [deg/s]/1 -> LateralController/6(Yaw rate [deg/s])
  vy [m/s]/1 -> LateralController/5(vy [m/s])
  vx [m/s]/1 -> LateralController/4(vx [m/s])
  position x,y,Y [m,m,deg]/1 -> LateralController/3(position x,y,Y [m,m,deg])
  ActorOffset_Left(+) / Right(-) [m]/1 -> LateralController/2(ActorOffset_Left(+) / Right(-) [m])
  TrajOffset x,y,Y [m,m,deg]/1 -> LateralController/1(TrajOffset x,y,Y [m,m,deg])
  LateralController/2(Actor/Traj_angle [deg]) -> Actor/Traj_angle [deg]/1
  LateralController/1(Actor/Traj_distance [m]) -> Actor/Traj_distance [m]/1
  velocity [m/s]/1 -> LongitudinalController/1(v_actual [m/s])
  LongitudinalController/1(throttle [%]) -> throttle [%]/1
  Desired Velocity [m/s]/1 -> LongitudinalController/2(Desired Velocity [m/s])
  Initial Velocity [m/s]/1 -> LongitudinalController/3(Initial Velocity [m/s])
  LongitudinalController/2(brake pressure [bar]) -> brake pressure [bar]/1
  LongitudinalController/3(v0 [m/s]) -> v0 [m/s]/1
  LongitudinalController/4(Auto_GearShift) -> Auto_GearShift/1

== system MCity_cs/Audi_A8_1/SELF_Demux ==
  SELF : Inport
  Demux1 : Demux  Outputs=3
  Demux2 : Demux  Outputs=3
  Demux3 : Demux  Outputs=[3 3 1 1]
  Demux4 : Demux  Outputs=3
  Gain : Gain  Gain=180/pi
  Gain1 : Gain  Gain=180/pi
  Selector : Selector  InputPortWidth=3  IndexOptions=Index vector (dialog)  Indices=[3]  OutputSizes=1
  compas converter : Subsystem
  xyz2GPS : PreScanUsefulBlocks/xyz2GPS  CoordinateCount=1  GPS_base=[0.000000 0.000000 0.000]
  x [m] : Outport
  y [m] : Outport  Port=2
  z [m] : Outport  Port=3
  rotx [deg] : Outport  Port=4
  roty [deg] : Outport  Port=5
  rotz [deg] : Outport  Port=6
  GPS lat [deg] : Outport  Port=7
  GPS long [deg] : Outport  Port=8
  GPS alt [m] : Outport  Port=9
  velocity [m/s] : Outport  Port=10
  heading [deg] : Outport  Port=11
  yaw rate [deg/s] : Outport  Port=12
  wires:
  Demux3/4 -> Gain1/1
  Gain1/1 -> yaw rate [deg/s]/1
  Demux3/3 -> velocity [m/s]/1
  compas converter/1(heading [deg]) -> heading [deg]/1
  xyz2GPS/1 -> Demux4/1
  Demux4/3 -> GPS alt [m]/1
  Demux4/2 -> GPS long [deg]/1
  Demux4/1 -> GPS lat [deg]/1
  Demux3/2 -> Gain/1, Selector/1
  Demux3/1 -> xyz2GPS/1, Demux1/1
  SELF/1 -> Demux3/1
  Demux2/3 -> rotz [deg]/1
  Demux2/2 -> roty [deg]/1
  Demux2/1 -> rotx [deg]/1
  Demux1/3 -> z [m]/1
  Demux1/2 -> y [m]/1
  Demux1/1 -> x [m]/1
  Gain/1 -> Demux2/1
  Selector/1 -> compas converter/1(rotz [rad])
